simulink model "rr_arm_control"  (R2026a)
settings: Solver=VariableStepAuto  MaxStep=1E-03
InitFcn:
  | rr_arm_control_init;
values from neighbouring files (symbols this model uses):
  b1 = 0.9    [rr_arm_control_init.m]
  b2 = 0.9    [rr_arm_control_init.m]
  g = 9.81    [rr_arm_control_init.m]
  G1 = blkdiag(diag([Ixx1,Iyy1,Izz1]),m1*eye(3))    [rr_arm_control_init.m]
  G2 = blkdiag(diag([Ixx2,Iyy2,Izz2]),m2*eye(3))    [rr_arm_control_init.m]
  M1 = [ ... (first row only)    [rr_arm_control_init.m]
  M2 = [ ... (first row only)    [rr_arm_control_init.m]
  params = [Iyy1,Iyy2,m1,m2,l1,l2,b1,b2,g].'    [rr_arm_control_init.m]
  S1 = rscrew('y',[0,0,0])    [rr_arm_control_init.m]
  S2 = rscrew('y',[l1,0,0])    [rr_arm_control_init.m]
(part 1 of 2)
settings Model: Creator=marti  LastModifiedBy=marti
settings SimscapeCC: SimscapeNominalValues="[{\"value\":\"1\",\"unit\":\"A\"},{\"value\":\"1\",\"unit\":\"bar\"},{\"value\":\"1\",\"unit\":\"cm^2\"},{\"value\":\"1\",\"unit\":\"cm^3/s\"},{\"value\":\"1\",\"unit\":\"kJ/kg\"},{\"value\":\"1\",\"unit\":\"kW\"},{\"value\":\"1\",\"unit\":\"l\"},{\"value\":\"1\",\"unit\":\"N\"},{\"value\":\"1\",\"unit\":\"N*m\"},{\"value\":\"1\",\"unit\":\"V\"}]"  SimscapeLogType=none  SimscapeLogDataHistory=5000.0

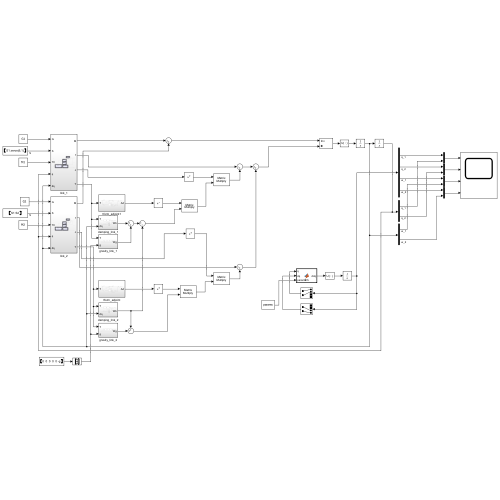
[thumbnail: Simulink's stored preview of the top-level diagram]
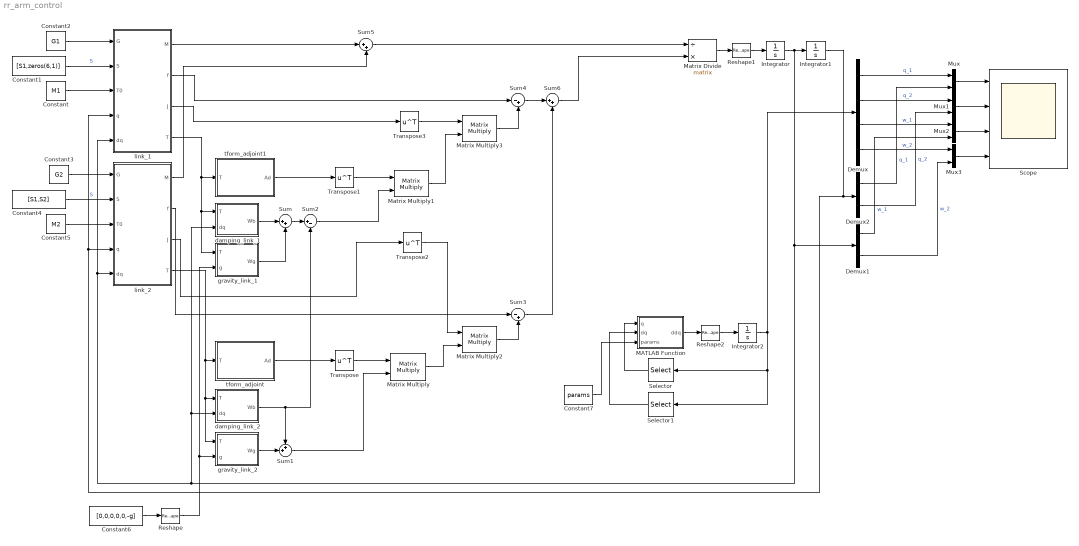
== system rr_arm_control ==
  Constant : Constant  Value=M1
  Constant1 : Constant  Value=[S1,zeros(6,1)]
  Constant2 : Constant  Value=G1
  Constant3 : Constant  Value=G2
  Constant4 : Constant  Value=[S1,S2]
  Constant5 : Constant  Value=M2
  Constant6 : Constant  Value=[0,0,0,0,0,-g]
  Constant7 : Constant  Value=params
  Demux : Demux
  Demux1 : Demux  Outputs=2
  Demux2 : Demux  Outputs=2
  Integrator : Integrator
  Integrator1 : Integrator  WrappedStateUpperValue=[pi,pi]'  WrappedStateLowerValue=-[pi,pi]'
  Integrator2 : Integrator
  MATLAB Function : MATLAB Function  TreatAsAtomicUnit=on
  Matrix Divide : Product  Inputs=/*  Multiplication=Matrix(*)
  Matrix Multiply{,1..3} (4 alike) : Product  Multiplication=Matrix(*)
  Mux{,1..3} (4 alike) : Mux  Inputs=2
  Reshape : Reshape  OutputDimensionality=Column vector (2-D)
  Reshape1 : Reshape
  Reshape2 : Reshape
  Scope : Scope  NumInputPorts=4
      settings: Title=q_1  ActiveDisplayYMinimum=-0.36221753295420889  ActiveDisplayYMaximum=3.2599577965878805  YLabel=angle (rad)
  Selector : Selector  InputPortWidth=4  IndexOptions=Index vector (dialog)  Indices=1:2  OutputSizes=1
  Selector1 : Selector  InputPortWidth=4  IndexOptions=Index vector (dialog)  Indices=3:4  OutputSizes=1
  Sum : Sum  Inputs=|++
  Sum1 : Sum  Inputs=++|
  Sum2 : Sum  Inputs=|+-
  Sum3 : Sum  Inputs=|-+
  Sum4 : Sum  Inputs=|-+
  Sum5 : Sum  Inputs=|++
  Sum6 : Sum  Inputs=|++
  Transpose{,1..3} (4 alike) : Math  Operator=transpose
  damping_link_1 : Subsystem
  damping_link_2 : Subsystem
  gravity_link_1 : Subsystem
  gravity_link_2 : Subsystem
  link_1 : Subsystem
  link_2 : Subsystem
  tform_adjoint : Subsystem
  tform_adjoint1 : Subsystem
  wires:
  Demux/1 -> Mux/1  "q_1"
  Demux2/1 -> Mux/2  "q_1"
  Demux/2 -> Mux1/1  "q_2"
  Demux2/2 -> Mux1/2  "q_2"
  Demux/3 -> Mux2/1  "w_1"
  Demux1/1 -> Mux2/2  "w_1"
  Demux/4 -> Mux3/1  "w_2"
  Demux1/2 -> Mux3/2  "w_2"
  Mux3/1 -> Scope/4
  Mux2/1 -> Scope/3
  Mux1/1 -> Scope/2
  Mux/1 -> Scope/1
  Constant2/1 -> link_1/1(G)
  Constant1/1 -> link_1/2(S)  "S"
  Constant/1 -> link_1/3(T0)
  Constant3/1 -> link_2/1(G)
  Constant4/1 -> link_2/2(S)  "S"
  Constant5/1 -> link_2/3(T0)
  Constant6/1 -> Reshape/1
  Matrix Divide/1 -> Reshape1/1
  Integrator/1 -> Integrator1/1, damping_link_2/2(dq), damping_link_1/2(dq), link_1/5(dq), link_2/5(dq), Demux1/1
  Reshape1/1 -> Integrator/1
  Integrator1/1 -> Demux2/1, link_1/4(q), link_2/4(q)
  MATLAB Function/1(ddq) -> Reshape2/1
  Reshape2/1 -> Integrator2/1
  Integrator2/1 -> Selector/1, Selector1/1, Demux/1
  Constant7/1 -> MATLAB Function/3(params)
  Selector/1 -> MATLAB Function/1(q)
  Selector1/1 -> MATLAB Function/2(dq)
  tform_adjoint/1(Ad) -> Transpose/1
  Transpose/1 -> Matrix Multiply/1
  Transpose1/1 -> Matrix Multiply1/1
  tform_adjoint1/1(Ad) -> Transpose1/1
  Transpose2/1 -> Matrix Multiply2/1
  Matrix Multiply/1 -> Matrix Multiply2/2
  Transpose3/1 -> Matrix Multiply3/1
  Matrix Multiply1/1 -> Matrix Multiply3/2
  link_1/4(T) -> gravity_link_1/1(T), damping_link_1/1(T), tform_adjoint1/1(T)
  Reshape/1 -> gravity_link_2/2(g), gravity_link_1/2(g)
  link_2/4(T) -> gravity_link_2/1(T), damping_link_2/1(T), tform_adjoint/1(T)
  damping_link_1/1(Wb) -> Sum/1
  gravity_link_1/1(Wg) -> Sum/2
  damping_link_2/1(Wb) -> Sum2/2, Sum1/1
  gravity_link_2/1(Wg) -> Sum1/2
  Sum/1 -> Sum2/1
  Sum1/1 -> Matrix Multiply/2
  link_2/3(J) -> Transpose2/1
  link_2/2(f) -> Sum3/1
  Matrix Multiply2/1 -> Sum3/2
  link_1/3(J) -> Transpose3/1
  Sum2/1 -> Matrix Multiply1/2
  Matrix Multiply3/1 -> Sum4/2
  link_1/2(f) -> Sum4/1
  link_1/1(M) -> Sum5/1
  link_2/1(M) -> Sum5/2
  Sum5/1 -> Matrix Divide/1
  Sum4/1 -> Sum6/1
  Sum3/1 -> Sum6/2
  Sum6/1 -> Matrix Divide/2

== system rr_arm_control/damping_link_1 ==
  T : Inport
  dq : Inport  Port=2
  Constant : Constant  Value=0
  Gain : Gain  Gain=-b1
  Matrix Multiply1 : Product  Multiplication=Matrix(*)
  Mux : Mux  Inputs=6
  Selector : Selector  InputPortWidth=2  IndexOptions=Index vector (dialog)  Indices=1  OutputSizes=1
  Transpose1 : Math  Operator=transpose
  tform_adjoint : Subsystem
  tform_inverse : Subsystem
  Wb : Outport
  wires:
  Matrix Multiply1/1 -> Wb/1
  tform_inverse/1(Tinv) -> tform_adjoint/1(T)
  tform_adjoint/1(Ad) -> Transpose1/1
  Transpose1/1 -> Matrix Multiply1/1
  T/1 -> tform_inverse/1(T)
  dq/1 -> Selector/1
  Selector/1 -> Gain/1
  Constant/1 -> Mux/6, Mux/5, Mux/4, Mux/3, Mux/1
  Gain/1 -> Mux/2
  Mux/1 -> Matrix Multiply1/2

== system rr_arm_control/damping_link_2 ==
  T : Inport
  dq : Inport  Port=2
  Constant : Constant  Value=0
  Gain : Gain  Gain=-b2
  Matrix Multiply1 : Product  Multiplication=Matrix(*)
  Mux : Mux  Inputs=6
  Selector : Selector  InputPortWidth=2  IndexOptions=Index vector (dialog)  Indices=2  OutputSizes=1
  Transpose1 : Math  Operator=transpose
  tform_adjoint : Subsystem
  tform_inverse : Subsystem
  Wb : Outport
  wires:
  Matrix Multiply1/1 -> Wb/1
  tform_inverse/1(Tinv) -> tform_adjoint/1(T)
  tform_adjoint/1(Ad) -> Transpose1/1
  Transpose1/1 -> Matrix Multiply1/1
  T/1 -> tform_inverse/1(T)
  dq/1 -> Selector/1
  Selector/1 -> Gain/1
  Constant/1 -> Mux/6, Mux/5, Mux/4, Mux/3, Mux/1
  Gain/1 -> Mux/2
  Mux/1 -> Matrix Multiply1/2

== system rr_arm_control/gravity_link_1 ==
  T : Inport
  g : Inport  Port=2
  Constant : Constant  Value=eye(3)
  Matrix Multiply1 : Product  Multiplication=Matrix(*)
  Selector : Selector  NumberOfDimensions=2  InputPortWidth=3  IndexOptions=Index vector (dialog),Index vector (dialog)  Indices=1:3,4  OutputSizes=1,1
  Transpose1 : Math  Operator=transpose
  tform : Subsystem
  tform_adjoint : Subsystem
  tform_inverse : Subsystem
  Wg : Outport
  wires:
  Matrix Multiply1/1 -> Wg/1
  T/1 -> Selector/1
  Selector/1 -> tform/2(p)
  Constant/1 -> tform/1(R)
  tform_inverse/1(Tinv) -> tform_adjoint/1(T)
  tform/1(T) -> tform_inverse/1(T)
  tform_adjoint/1(Ad) -> Transpose1/1
  Transpose1/1 -> Matrix Multiply1/1
  g/1 -> Matrix Multiply1/2

== system rr_arm_control/gravity_link_2 ==
  T : Inport
  g : Inport  Port=2
  Constant : Constant  Value=eye(3)
  Matrix Multiply1 : Product  Multiplication=Matrix(*)
  Selector : Selector  NumberOfDimensions=2  InputPortWidth=3  IndexOptions=Index vector (dialog),Index vector (dialog)  Indices=1:3,4  OutputSizes=1,1
  Transpose1 : Math  Operator=transpose
  tform : Subsystem
  tform_adjoint : Subsystem
  tform_inverse : Subsystem
  Wg : Outport
  wires:
  Matrix Multiply1/1 -> Wg/1
  T/1 -> Selector/1
  Selector/1 -> tform/2(p)
  Constant/1 -> tform/1(R)
  tform_inverse/1(Tinv) -> tform_adjoint/1(T)
  tform/1(T) -> tform_inverse/1(T)
  tform_adjoint/1(Ad) -> Transpose1/1
  Transpose1/1 -> Matrix Multiply1/1
  g/1 -> Matrix Multiply1/2

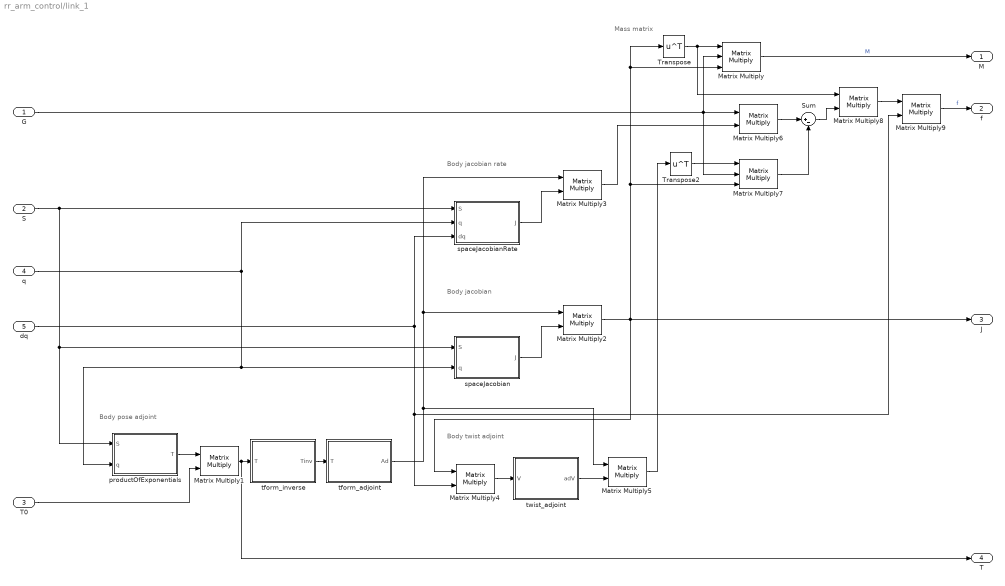
== system rr_arm_control/link_1 ==
  note: Body jacobian
  note: Body twist adjoint
  note: Mass matrix
  note: Body jacobian rate
  note: Body pose adjoint
  G : Inport
  S : Inport  Port=2
  T0 : Inport  Port=3
  q : Inport  Port=4
  dq : Inport  Port=5
  Matrix Multiply : Product  Inputs=3  Multiplication=Matrix(*)
  Matrix Multiply{1..6,8..9} (8 alike) : Product  Multiplication=Matrix(*)
  Matrix Multiply7 : Product  Inputs=3  Multiplication=Matrix(*)
  Sum : Sum  Inputs=|+-
  Transpose : Math  Operator=transpose
  Transpose2 : Math  Operator=transpose
  productOfExponentials : Subsystem  TreatAsAtomicUnit=on
  spaceJacobian : Subsystem  TreatAsAtomicUnit=on
  spaceJacobianRate : Subsystem  TreatAsAtomicUnit=on
  tform_adjoint : Subsystem
  tform_inverse : Subsystem
  twist_adjoint : Subsystem
  M : Outport
  f : Outport  Port=2
  J : Outport  Port=3
  T : Outport  Port=4
  wires:
  Matrix Multiply3/1 -> Matrix Multiply6/2
  Matrix Multiply2/1 -> Matrix Multiply7/3, Matrix Multiply/3, Transpose/1, J/1, Matrix Multiply4/1
  S/1 -> productOfExponentials/1(S), spaceJacobian/1(S), spaceJacobianRate/1(S)
  Matrix Multiply6/1 -> Sum/1
  G/1 -> Matrix Multiply6/1, Matrix Multiply7/2, Matrix Multiply/2
  twist_adjoint/1(adV) -> Matrix Multiply5/2
  Transpose/1 -> Matrix Multiply8/1, Matrix Multiply/1
  productOfExponentials/1(T) -> Matrix Multiply1/1
  spaceJacobian/1(J) -> Matrix Multiply2/2
  tform_inverse/1(Tinv) -> tform_adjoint/1(T)
  Matrix Multiply8/1 -> Matrix Multiply9/1
  tform_adjoint/1(Ad) -> Matrix Multiply3/1, Matrix Multiply2/1, Matrix Multiply5/1
  Matrix Multiply5/1 -> Transpose2/1
  q/1 -> spaceJacobian/2(q), productOfExponentials/2(q), spaceJacobianRate/2(q)
  Matrix Multiply1/1 -> T/1, tform_inverse/1(T)
  Matrix Multiply7/1 -> Sum/2
  Sum/1 -> Matrix Multiply8/2
  Matrix Multiply/1 -> M/1  "M"
  spaceJacobianRate/1(J) -> Matrix Multiply3/2
  Matrix Multiply4/1 -> twist_adjoint/1(V)
  T0/1 -> Matrix Multiply1/2
  dq/1 -> Matrix Multiply9/2, Matrix Multiply4/2, spaceJacobianRate/3(dq)
  Matrix Multiply9/1 -> f/1  "f"
  Transpose2/1 -> Matrix Multiply7/1

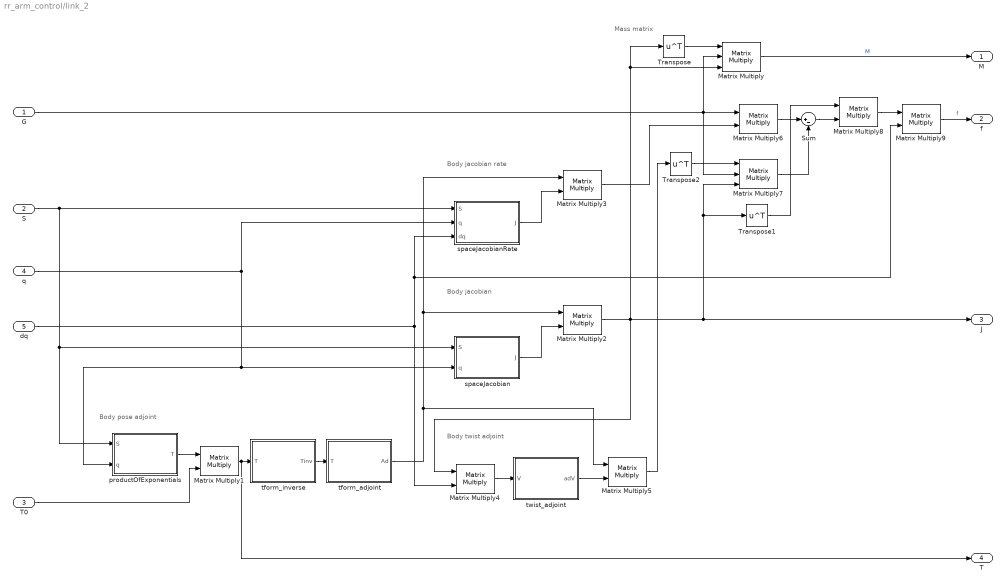
== system rr_arm_control/link_2 ==
  note: Body jacobian
  note: Body twist adjoint
  note: Mass matrix
  note: Body jacobian rate
  note: Body pose adjoint
  G : Inport
  S : Inport  Port=2
  T0 : Inport  Port=3
  q : Inport  Port=4
  dq : Inport  Port=5
  Matrix Multiply : Product  Inputs=3  Multiplication=Matrix(*)
  Matrix Multiply{1..6,8..9} (8 alike) : Product  Multiplication=Matrix(*)
  Matrix Multiply7 : Product  Inputs=3  Multiplication=Matrix(*)
  Sum : Sum  Inputs=|+-
  Transpose : Math  Operator=transpose
  Transpose1 : Math  Operator=transpose
  Transpose2 : Math  Operator=transpose
  productOfExponentials : Subsystem  TreatAsAtomicUnit=on
  spaceJacobian : Subsystem  TreatAsAtomicUnit=on
  spaceJacobianRate : Subsystem  TreatAsAtomicUnit=on
  tform_adjoint : Subsystem
  tform_inverse : Subsystem
  twist_adjoint : Subsystem
  M : Outport
  f : Outport  Port=2
  J : Outport  Port=3
  T : Outport  Port=4
  wires:
  Matrix Multiply3/1 -> Matrix Multiply6/2
  Matrix Multiply2/1 -> J/1, Transpose1/1, Matrix Multiply7/3, Matrix Multiply4/1, Matrix Multiply/3, Transpose/1
  S/1 -> productOfExponentials/1(S), spaceJacobian/1(S), spaceJacobianRate/1(S)
  Matrix Multiply6/1 -> Sum/1
  Transpose1/1 -> Matrix Multiply8/1
  G/1 -> Matrix Multiply6/1, Matrix Multiply7/2, Matrix Multiply/2
  twist_adjoint/1(adV) -> Matrix Multiply5/2
  Transpose/1 -> Matrix Multiply/1
  productOfExponentials/1(T) -> Matrix Multiply1/1
  spaceJacobian/1(J) -> Matrix Multiply2/2
  tform_inverse/1(Tinv) -> tform_adjoint/1(T)
  Matrix Multiply8/1 -> Matrix Multiply9/1
  tform_adjoint/1(Ad) -> Matrix Multiply3/1, Matrix Multiply2/1, Matrix Multiply5/1
  Matrix Multiply5/1 -> Transpose2/1
  q/1 -> spaceJacobian/2(q), productOfExponentials/2(q), spaceJacobianRate/2(q)
  Matrix Multiply1/1 -> T/1, tform_inverse/1(T)
  Matrix Multiply7/1 -> Sum/2
  Sum/1 -> Matrix Multiply8/2
  Matrix Multiply/1 -> M/1  "M"
  spaceJacobianRate/1(J) -> Matrix Multiply3/2
  Matrix Multiply4/1 -> twist_adjoint/1(V)
  T0/1 -> Matrix Multiply1/2
  dq/1 -> spaceJacobianRate/3(dq), Matrix Multiply9/2, Matrix Multiply4/2
  Matrix Multiply9/1 -> f/1  "f"
  Transpose2/1 -> Matrix Multiply7/1

== system rr_arm_control/tform_adjoint ==
  T : Inport
  Constant : Constant  Value=zeros(3)
  Matrix Concatenate : Concatenate  Mode=Multidimensional array  ConcatenateDimension=2
  Matrix Concatenate1 : Concatenate  Mode=Multidimensional array  ConcatenateDimension=2
  Matrix Concatenate2 : Concatenate  Mode=Multidimensional array
  Matrix Multiply : Product  Multiplication=Matrix(*)
  Selector : Selector  NumberOfDimensions=2  InputPortWidth=3  IndexOptions=Index vector (dialog),Index vector (dialog)  Indices=1:3,1:3  OutputSizes=1,1
  Selector1 : Selector  NumberOfDimensions=2  InputPortWidth=3  IndexOptions=Index vector (dialog),Index vector (dialog)  Indices=1:3,4  OutputSizes=1,1
  vec2skew : Subsystem
  Ad : Outport
  wires:
  Selector1/1 -> vec2skew/1(x)
  Selector/1 -> Matrix Multiply/2, Matrix Concatenate1/2, Matrix Concatenate/1
  Constant/1 -> Matrix Concatenate/2
  vec2skew/1("[x]") -> Matrix Multiply/1
  Matrix Multiply/1 -> Matrix Concatenate1/1
  Matrix Concatenate1/1 -> Matrix Concatenate2/2
  Matrix Concatenate/1 -> Matrix Concatenate2/1
  Matrix Concatenate2/1 -> Ad/1
  T/1 -> Selector1/1, Selector/1

== system rr_arm_control/tform_adjoint1 ==
  T : Inport
  Constant : Constant  Value=zeros(3)
  Matrix Concatenate : Concatenate  Mode=Multidimensional array  ConcatenateDimension=2
  Matrix Concatenate1 : Concatenate  Mode=Multidimensional array  ConcatenateDimension=2
  Matrix Concatenate2 : Concatenate  Mode=Multidimensional array
  Matrix Multiply : Product  Multiplication=Matrix(*)
  Selector : Selector  NumberOfDimensions=2  InputPortWidth=3  IndexOptions=Index vector (dialog),Index vector (dialog)  Indices=1:3,1:3  OutputSizes=1,1
  Selector1 : Selector  NumberOfDimensions=2  InputPortWidth=3  IndexOptions=Index vector (dialog),Index vector (dialog)  Indices=1:3,4  OutputSizes=1,1
  vec2skew : Subsystem
  Ad : Outport
  wires:
  Selector1/1 -> vec2skew/1(x)
  Selector/1 -> Matrix Multiply/2, Matrix Concatenate1/2, Matrix Concatenate/1
  Constant/1 -> Matrix Concatenate/2
  vec2skew/1("[x]") -> Matrix Multiply/1
  Matrix Multiply/1 -> Matrix Concatenate1/1
  Matrix Concatenate1/1 -> Matrix Concatenate2/2
  Matrix Concatenate/1 -> Matrix Concatenate2/1
  Matrix Concatenate2/1 -> Ad/1
  T/1 -> Selector1/1, Selector/1

== system rr_arm_control/damping_link_1/tform_adjoint ==
  T : Inport
  Constant : Constant  Value=zeros(3)
  Matrix Concatenate : Concatenate  Mode=Multidimensional array  ConcatenateDimension=2
  Matrix Concatenate1 : Concatenate  Mode=Multidimensional array  ConcatenateDimension=2
  Matrix Concatenate2 : Concatenate  Mode=Multidimensional array
  Matrix Multiply : Product  Multiplication=Matrix(*)
  Selector : Selector  NumberOfDimensions=2  InputPortWidth=3  IndexOptions=Index vector (dialog),Index vector (dialog)  Indices=1:3,1:3  OutputSizes=1,1
  Selector1 : Selector  NumberOfDimensions=2  InputPortWidth=3  IndexOptions=Index vector (dialog),Index vector (dialog)  Indices=1:3,4  OutputSizes=1,1
  vec2skew : Subsystem
  Ad : Outport
  wires:
  Selector1/1 -> vec2skew/1(x)
  Selector/1 -> Matrix Multiply/2, Matrix Concatenate1/2, Matrix Concatenate/1
  Constant/1 -> Matrix Concatenate/2
  vec2skew/1("[x]") -> Matrix Multiply/1
  Matrix Multiply/1 -> Matrix Concatenate1/1
  Matrix Concatenate1/1 -> Matrix Concatenate2/2
  Matrix Concatenate/1 -> Matrix Concatenate2/1
  Matrix Concatenate2/1 -> Ad/1
  T/1 -> Selector1/1, Selector/1

== system rr_arm_control/damping_link_1/tform_inverse ==
  T : Inport
  Constant : Constant  Value=[0,0,0,1]
  Gain : Gain  Gain=-1
  Matrix Concatenate : Concatenate  Mode=Multidimensional array  ConcatenateDimension=2
  Matrix Concatenate1 : Concatenate  Mode=Multidimensional array
  Matrix Multiply : Product  Multiplication=Matrix(*)
  Reshape : Reshape  OutputDimensionality=Row vector (2-D)
  Selector : Selector  NumberOfDimensions=2  InputPortWidth=3  IndexOptions=Index vector (dialog),Index vector (dialog)  Indices=1:3,1:3  OutputSizes=1,1
  Selector1 : Selector  NumberOfDimensions=2  InputPortWidth=3  IndexOptions=Index vector (dialog),Index vector (dialog)  Indices=1:3,4  OutputSizes=1,1
  Transpose : Math  Operator=transpose
  Tinv : Outport
  wires:
  T/1 -> Selector1/1, Selector/1
  Selector/1 -> Transpose/1
  Transpose/1 -> Matrix Multiply/1, Matrix Concatenate/1
  Matrix Multiply/1 -> Gain/1
  Gain/1 -> Matrix Concatenate/2
  Matrix Concatenate/1 -> Matrix Concatenate1/1
  Constant/1 -> Reshape/1
  Matrix Concatenate1/1 -> Tinv/1
  Selector1/1 -> Matrix Multiply/2
  Reshape/1 -> Matrix Concatenate1/2

== system rr_arm_control/damping_link_2/tform_adjoint ==
  T : Inport
  Constant : Constant  Value=zeros(3)
  Matrix Concatenate : Concatenate  Mode=Multidimensional array  ConcatenateDimension=2
  Matrix Concatenate1 : Concatenate  Mode=Multidimensional array  ConcatenateDimension=2
  Matrix Concatenate2 : Concatenate  Mode=Multidimensional array
  Matrix Multiply : Product  Multiplication=Matrix(*)
  Selector : Selector  NumberOfDimensions=2  InputPortWidth=3  IndexOptions=Index vector (dialog),Index vector (dialog)  Indices=1:3,1:3  OutputSizes=1,1
  Selector1 : Selector  NumberOfDimensions=2  InputPortWidth=3  IndexOptions=Index vector (dialog),Index vector (dialog)  Indices=1:3,4  OutputSizes=1,1
  vec2skew : Subsystem
  Ad : Outport
  wires:
  Selector1/1 -> vec2skew/1(x)
  Selector/1 -> Matrix Multiply/2, Matrix Concatenate1/2, Matrix Concatenate/1
  Constant/1 -> Matrix Concatenate/2
  vec2skew/1("[x]") -> Matrix Multiply/1
  Matrix Multiply/1 -> Matrix Concatenate1/1
  Matrix Concatenate1/1 -> Matrix Concatenate2/2
  Matrix Concatenate/1 -> Matrix Concatenate2/1
  Matrix Concatenate2/1 -> Ad/1
  T/1 -> Selector1/1, Selector/1

== system rr_arm_control/damping_link_2/tform_inverse ==
  T : Inport
  Constant : Constant  Value=[0,0,0,1]
  Gain : Gain  Gain=-1
  Matrix Concatenate : Concatenate  Mode=Multidimensional array  ConcatenateDimension=2
  Matrix Concatenate1 : Concatenate  Mode=Multidimensional array
  Matrix Multiply : Product  Multiplication=Matrix(*)
  Reshape : Reshape  OutputDimensionality=Row vector (2-D)
  Selector : Selector  NumberOfDimensions=2  InputPortWidth=3  IndexOptions=Index vector (dialog),Index vector (dialog)  Indices=1:3,1:3  OutputSizes=1,1
  Selector1 : Selector  NumberOfDimensions=2  InputPortWidth=3  IndexOptions=Index vector (dialog),Index vector (dialog)  Indices=1:3,4  OutputSizes=1,1
  Transpose : Math  Operator=transpose
  Tinv : Outport
  wires:
  T/1 -> Selector1/1, Selector/1
  Selector/1 -> Transpose/1
  Transpose/1 -> Matrix Multiply/1, Matrix Concatenate/1
  Matrix Multiply/1 -> Gain/1
  Gain/1 -> Matrix Concatenate/2
  Matrix Concatenate/1 -> Matrix Concatenate1/1
  Constant/1 -> Reshape/1
  Matrix Concatenate1/1 -> Tinv/1
  Selector1/1 -> Matrix Multiply/2
  Reshape/1 -> Matrix Concatenate1/2

== system rr_arm_control/gravity_link_1/tform ==
  R : Inport
  p : Inport  Port=2
  Constant : Constant  Value=[0,0,0,1]
  Matrix Concatenate : Concatenate  Mode=Multidimensional array  ConcatenateDimension=2
  Matrix Concatenate2 : Concatenate  Mode=Multidimensional array
  Reshape : Reshape  OutputDimensionality=Row vector (2-D)
  T : Outport
  wires:
  p/1 -> Matrix Concatenate/2
  Constant/1 -> Reshape/1
  Matrix Concatenate/1 -> Matrix Concatenate2/1
  Matrix Concatenate2/1 -> T/1
  R/1 -> Matrix Concatenate/1
  Reshape/1 -> Matrix Concatenate2/2

== system rr_arm_control/gravity_link_1/tform_adjoint ==
  T : Inport
  Constant : Constant  Value=zeros(3)
  Matrix Concatenate : Concatenate  Mode=Multidimensional array  ConcatenateDimension=2
  Matrix Concatenate1 : Concatenate  Mode=Multidimensional array  ConcatenateDimension=2
  Matrix Concatenate2 : Concatenate  Mode=Multidimensional array
  Matrix Multiply : Product  Multiplication=Matrix(*)
  Selector : Selector  NumberOfDimensions=2  InputPortWidth=3  IndexOptions=Index vector (dialog),Index vector (dialog)  Indices=1:3,1:3  OutputSizes=1,1
  Selector1 : Selector  NumberOfDimensions=2  InputPortWidth=3  IndexOptions=Index vector (dialog),Index vector (dialog)  Indices=1:3,4  OutputSizes=1,1
  vec2skew : Subsystem
  Ad : Outport
  wires:
  Selector1/1 -> vec2skew/1(x)
  Selector/1 -> Matrix Multiply/2, Matrix Concatenate1/2, Matrix Concatenate/1
  Constant/1 -> Matrix Concatenate/2
  vec2skew/1("[x]") -> Matrix Multiply/1
  Matrix Multiply/1 -> Matrix Concatenate1/1
  Matrix Concatenate1/1 -> Matrix Concatenate2/2
  Matrix Concatenate/1 -> Matrix Concatenate2/1
  Matrix Concatenate2/1 -> Ad/1
  T/1 -> Selector1/1, Selector/1

== system rr_arm_control/gravity_link_1/tform_inverse ==
  T : Inport
  Constant : Constant  Value=[0,0,0,1]
  Gain : Gain  Gain=-1
  Matrix Concatenate : Concatenate  Mode=Multidimensional array  ConcatenateDimension=2
  Matrix Concatenate1 : Concatenate  Mode=Multidimensional array
  Matrix Multiply : Product  Multiplication=Matrix(*)
  Reshape : Reshape  OutputDimensionality=Row vector (2-D)
  Selector : Selector  NumberOfDimensions=2  InputPortWidth=3  IndexOptions=Index vector (dialog),Index vector (dialog)  Indices=1:3,1:3  OutputSizes=1,1
  Selector1 : Selector  NumberOfDimensions=2  InputPortWidth=3  IndexOptions=Index vector (dialog),Index vector (dialog)  Indices=1:3,4  OutputSizes=1,1
  Transpose : Math  Operator=transpose
  Tinv : Outport
  wires:
  T/1 -> Selector1/1, Selector/1
  Selector/1 -> Transpose/1
  Transpose/1 -> Matrix Multiply/1, Matrix Concatenate/1
  Matrix Multiply/1 -> Gain/1
  Gain/1 -> Matrix Concatenate/2
  Matrix Concatenate/1 -> Matrix Concatenate1/1
  Constant/1 -> Reshape/1
  Matrix Concatenate1/1 -> Tinv/1
  Selector1/1 -> Matrix Multiply/2
  Reshape/1 -> Matrix Concatenate1/2

== system rr_arm_control/gravity_link_2/tform ==
  R : Inport
  p : Inport  Port=2
  Constant : Constant  Value=[0,0,0,1]
  Matrix Concatenate : Concatenate  Mode=Multidimensional array  ConcatenateDimension=2
  Matrix Concatenate2 : Concatenate  Mode=Multidimensional array
  Reshape : Reshape  OutputDimensionality=Row vector (2-D)
  T : Outport
  wires:
  p/1 -> Matrix Concatenate/2
  Constant/1 -> Reshape/1
  Matrix Concatenate/1 -> Matrix Concatenate2/1
  Matrix Concatenate2/1 -> T/1
  R/1 -> Matrix Concatenate/1
  Reshape/1 -> Matrix Concatenate2/2

== system rr_arm_control/gravity_link_2/tform_adjoint ==
  T : Inport
  Constant : Constant  Value=zeros(3)
  Matrix Concatenate : Concatenate  Mode=Multidimensional array  ConcatenateDimension=2
  Matrix Concatenate1 : Concatenate  Mode=Multidimensional array  ConcatenateDimension=2
  Matrix Concatenate2 : Concatenate  Mode=Multidimensional array
  Matrix Multiply : Product  Multiplication=Matrix(*)
  Selector : Selector  NumberOfDimensions=2  InputPortWidth=3  IndexOptions=Index vector (dialog),Index vector (dialog)  Indices=1:3,1:3  OutputSizes=1,1
  Selector1 : Selector  NumberOfDimensions=2  InputPortWidth=3  IndexOptions=Index vector (dialog),Index vector (dialog)  Indices=1:3,4  OutputSizes=1,1
  vec2skew : Subsystem
  Ad : Outport
  wires:
  Selector1/1 -> vec2skew/1(x)
  Selector/1 -> Matrix Multiply/2, Matrix Concatenate1/2, Matrix Concatenate/1
  Constant/1 -> Matrix Concatenate/2
  vec2skew/1("[x]") -> Matrix Multiply/1
  Matrix Multiply/1 -> Matrix Concatenate1/1
  Matrix Concatenate1/1 -> Matrix Concatenate2/2
  Matrix Concatenate/1 -> Matrix Concatenate2/1
  Matrix Concatenate2/1 -> Ad/1
  T/1 -> Selector1/1, Selector/1

== system rr_arm_control/gravity_link_2/tform_inverse ==
  T : Inport
  Constant : Constant  Value=[0,0,0,1]
  Gain : Gain  Gain=-1
  Matrix Concatenate : Concatenate  Mode=Multidimensional array  ConcatenateDimension=2
  Matrix Concatenate1 : Concatenate  Mode=Multidimensional array
  Matrix Multiply : Product  Multiplication=Matrix(*)
  Reshape : Reshape  OutputDimensionality=Row vector (2-D)
  Selector : Selector  NumberOfDimensions=2  InputPortWidth=3  IndexOptions=Index vector (dialog),Index vector (dialog)  Indices=1:3,1:3  OutputSizes=1,1
  Selector1 : Selector  NumberOfDimensions=2  InputPortWidth=3  IndexOptions=Index vector (dialog),Index vector (dialog)  Indices=1:3,4  OutputSizes=1,1
  Transpose : Math  Operator=transpose
  Tinv : Outport
  wires:
  T/1 -> Selector1/1, Selector/1
  Selector/1 -> Transpose/1
  Transpose/1 -> Matrix Multiply/1, Matrix Concatenate/1
  Matrix Multiply/1 -> Gain/1
  Gain/1 -> Matrix Concatenate/2
  Matrix Concatenate/1 -> Matrix Concatenate1/1
  Constant/1 -> Reshape/1
  Matrix Concatenate1/1 -> Tinv/1
  Selector1/1 -> Matrix Multiply/2
  Reshape/1 -> Matrix Concatenate1/2

== system rr_arm_control/link_1/productOfExponentials ==
  S : Inport
  q : Inport  Port=2
  For Iterator : ForIterator  ResetStates=reset  IterationSource=external
  Matrix Multiply : Product  Multiplication=Matrix(*)
  Memory : Memory  InitialCondition=eye(4)  InheritSampleTime=on
  Probe Dimension : Probe  ProbeWidth=off  ProbeSampleTime=off  ProbeComplexSignal=off  ProbeSignalDimensions=on
  Reshape : Reshape  OutputDimensionality=Column vector (2-D)
  Selector : Selector  NumberOfDimensions=2  InputPortWidth=3  IndexOptions=Select all,Index vector (port)  Indices=[1 3],1  OutputSizes=1,1
  Selector1 : Selector  NumberOfDimensions=2  InputPortWidth=3  IndexOptions=Index vector (port),Select all  Indices=[1 3],1  OutputSizes=1,1
  Subsystem1 : Subsystem
  T : Outport
  wires:
  For Iterator/1 -> Selector1/2, Selector/2
  q/1 -> Reshape/1, Probe Dimension/1
  Probe Dimension/1 -> For Iterator/1
  S/1 -> Selector/1
  Selector/1 -> Subsystem1/1(S)
  Reshape/1 -> Selector1/1
  Selector1/1 -> Subsystem1/2(q)
  Subsystem1/1(T) -> Matrix Multiply/2
  Matrix Multiply/1 -> Memory/1, T/1
  Memory/1 -> Matrix Multiply/1

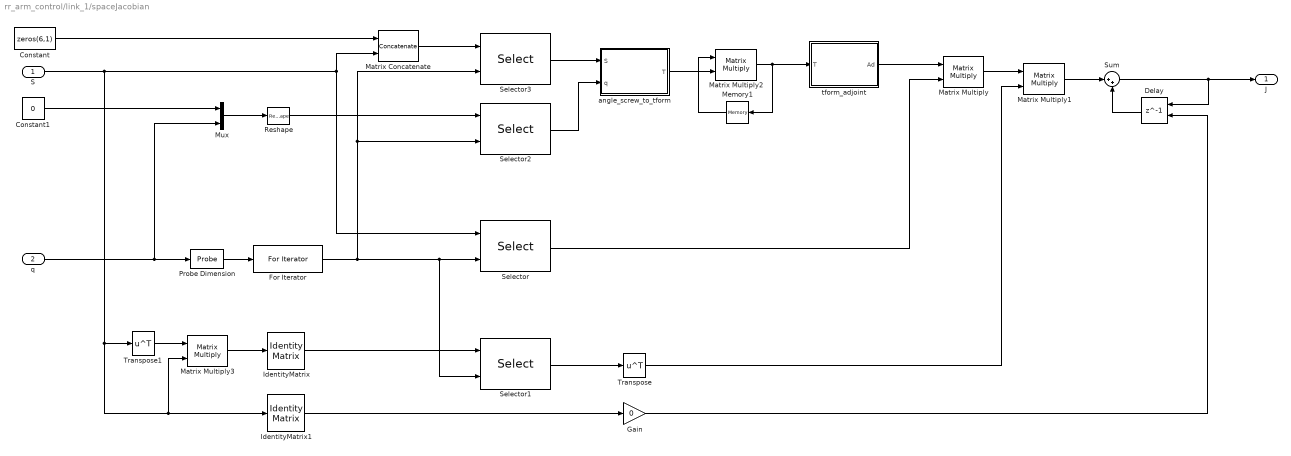
== system rr_arm_control/link_1/spaceJacobian ==
  S : Inport
  q : Inport  Port=2
  Constant : Constant  Value=zeros(6,1)
  Constant1 : Constant  Value=0
  Delay : Delay  DelayLength=1  InitialConditionSource=Input port
      settings: InputPortMap=u0,p4
  For Iterator : ForIterator  ResetStates=reset  IterationSource=external  IterationLimit=4
  Gain : Gain  Gain=0
  IdentityMatrix : IdentityMatrix  InheritOutputPortAttributes=on
  IdentityMatrix1 : IdentityMatrix  InheritOutputPortAttributes=on
  Matrix Concatenate : Concatenate  Mode=Multidimensional array  ConcatenateDimension=2
  Matrix Multiply{,1..3} (4 alike) : Product  Multiplication=Matrix(*)
  Memory1 : Memory  InitialCondition=eye(4)  InheritSampleTime=on
  Mux : Mux  Inputs=2
  Probe Dimension : Probe  ProbeWidth=off  ProbeSampleTime=off  ProbeComplexSignal=off  ProbeSignalDimensions=on
  Reshape : Reshape  OutputDimensionality=Column vector (2-D)
  Selector : Selector  NumberOfDimensions=2  InputPortWidth=3  IndexOptions=Select all,Index vector (port)  Indices=[1 3],1  OutputSizes=1,1
  Selector1 : Selector  NumberOfDimensions=2  InputPortWidth=3  IndexOptions=Select all,Index vector (port)  Indices=[1 3],1  OutputSizes=1,1
  Selector2 : Selector  NumberOfDimensions=2  InputPortWidth=3  IndexOptions=Index vector (port),Select all  Indices=[1 3],1  OutputSizes=1,1
  Selector3 : Selector  NumberOfDimensions=2  InputPortWidth=3  IndexOptions=Select all,Index vector (port)  Indices=[1 3],1  OutputSizes=1,1
  Sum : Sum  Inputs=|++
  Transpose : Math  Operator=transpose
  Transpose1 : Math  Operator=transpose
  angle_screw_to_tform : Subsystem
  tform_adjoint : Subsystem
  J : Outport
  wires:
  S/1 -> Matrix Concatenate/2, Selector/1, IdentityMatrix1/1, Matrix Multiply3/2, Transpose1/1
  Matrix Multiply1/1 -> Sum/1
  Sum/1 -> Delay/1, J/1
  tform_adjoint/1(Ad) -> Matrix Multiply/1
  Selector/1 -> Matrix Multiply/2
  For Iterator/1 -> Selector1/2, Selector/2, Selector3/2, Selector2/2
  Matrix Multiply/1 -> Matrix Multiply1/1
  Transpose/1 -> Matrix Multiply1/2
  angle_screw_to_tform/1(T) -> Matrix Multiply2/2
  Matrix Multiply2/1 -> tform_adjoint/1(T), Memory1/1
  Memory1/1 -> Matrix Multiply2/1
  Selector2/1 -> angle_screw_to_tform/2(q)
  Selector3/1 -> angle_screw_to_tform/1(S)
  IdentityMatrix/1 -> Selector1/1
  Selector1/1 -> Transpose/1
  q/1 -> Mux/2, Probe Dimension/1
  Matrix Multiply3/1 -> IdentityMatrix/1
  Transpose1/1 -> Matrix Multiply3/1
  IdentityMatrix1/1 -> Gain/1
  Gain/1 -> Delay/2
  Delay/1 -> Sum/2
  Probe Dimension/1 -> For Iterator/1
  Mux/1 -> Reshape/1
  Constant1/1 -> Mux/1
  Reshape/1 -> Selector2/1
  Matrix Concatenate/1 -> Selector3/1
  Constant/1 -> Matrix Concatenate/1

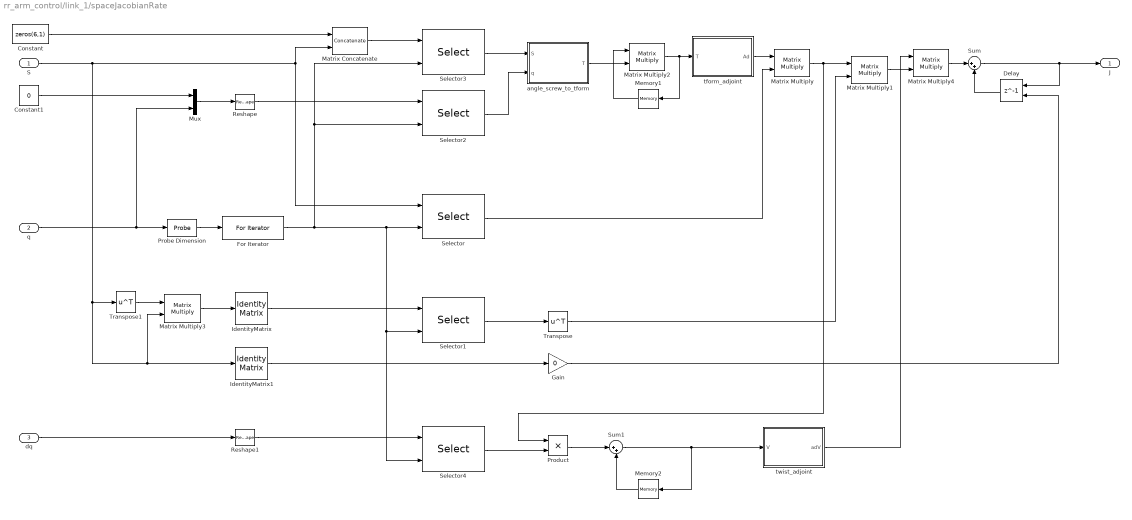
== system rr_arm_control/link_1/spaceJacobianRate ==
  S : Inport
  q : Inport  Port=2
  dq : Inport  Port=3
  Constant : Constant  Value=zeros(6,1)
  Constant1 : Constant  Value=0
  Delay : Delay  DelayLength=1  InitialConditionSource=Input port
      settings: InputPortMap=u0,p4
  For Iterator : ForIterator  ResetStates=reset  IterationSource=external  IterationLimit=4
  Gain : Gain  Gain=0
  IdentityMatrix : IdentityMatrix  InheritOutputPortAttributes=on
  IdentityMatrix1 : IdentityMatrix  InheritOutputPortAttributes=on
  Matrix Concatenate : Concatenate  Mode=Multidimensional array  ConcatenateDimension=2
  Matrix Multiply{,1..4} (5 alike) : Product  Multiplication=Matrix(*)
  Memory1 : Memory  InitialCondition=eye(4)  InheritSampleTime=on
  Memory2 : Memory  InitialCondition=zeros(6,1)  InheritSampleTime=on
  Mux : Mux  Inputs=2
  Probe Dimension : Probe  ProbeWidth=off  ProbeSampleTime=off  ProbeComplexSignal=off  ProbeSignalDimensions=on
  Product : Product
  Reshape : Reshape  OutputDimensionality=Column vector (2-D)
  Reshape1 : Reshape  OutputDimensionality=Column vector (2-D)
  Selector : Selector  NumberOfDimensions=2  InputPortWidth=3  IndexOptions=Select all,Index vector (port)  Indices=[1 3],1  OutputSizes=1,1
  Selector1 : Selector  NumberOfDimensions=2  InputPortWidth=3  IndexOptions=Select all,Index vector (port)  Indices=[1 3],1  OutputSizes=1,1
  Selector2 : Selector  NumberOfDimensions=2  InputPortWidth=3  IndexOptions=Index vector (port),Select all  Indices=[1 3],1  OutputSizes=1,1
  Selector3 : Selector  NumberOfDimensions=2  InputPortWidth=3  IndexOptions=Select all,Index vector (port)  Indices=[1 3],1  OutputSizes=1,1
  Selector4 : Selector  NumberOfDimensions=2  InputPortWidth=3  IndexOptions=Index vector (port),Select all  Indices=[1 3],1  OutputSizes=1,1
  Sum : Sum  Inputs=|++
  Sum1 : Sum  Inputs=|++
  Transpose : Math  Operator=transpose
  Transpose1 : Math  Operator=transpose
  angle_screw_to_tform : Subsystem
  tform_adjoint : Subsystem
  twist_adjoint : Subsystem
  J : Outport
  wires:
  S/1 -> Matrix Concatenate/2, Selector/1, IdentityMatrix1/1, Matrix Multiply3/2, Transpose1/1
  Sum/1 -> Delay/1, J/1
  tform_adjoint/1(Ad) -> Matrix Multiply/1
  Selector/1 -> Matrix Multiply/2
  For Iterator/1 -> Selector4/2, Selector1/2, Selector/2, Selector3/2, Selector2/2
  Matrix Multiply/1 -> Product/1, Matrix Multiply1/1
  Transpose/1 -> Matrix Multiply1/2
  angle_screw_to_tform/1(T) -> Matrix Multiply2/2
  Matrix Multiply2/1 -> tform_adjoint/1(T), Memory1/1
  Memory1/1 -> Matrix Multiply2/1
  Selector2/1 -> angle_screw_to_tform/2(q)
  Selector3/1 -> angle_screw_to_tform/1(S)
  IdentityMatrix/1 -> Selector1/1
  Selector1/1 -> Transpose/1
  q/1 -> Mux/2, Probe Dimension/1
  Matrix Multiply3/1 -> IdentityMatrix/1
  Transpose1/1 -> Matrix Multiply3/1
  IdentityMatrix1/1 -> Gain/1
  Gain/1 -> Delay/2
  Delay/1 -> Sum/2
  Probe Dimension/1 -> For Iterator/1
  Mux/1 -> Reshape/1
  Constant1/1 -> Mux/1
  Reshape/1 -> Selector2/1
  Matrix Concatenate/1 -> Selector3/1
  Constant/1 -> Matrix Concatenate/1
  Matrix Multiply1/1 -> Matrix Multiply4/2
  Matrix Multiply4/1 -> Sum/1
  dq/1 -> Reshape1/1
  Reshape1/1 -> Selector4/1
  Selector4/1 -> Product/2
  Product/1 -> Sum1/1
  Memory2/1 -> Sum1/2
  Sum1/1 -> Memory2/1, twist_adjoint/1(V)
  twist_adjoint/1(adV) -> Matrix Multiply4/1

== system rr_arm_control/link_1/tform_adjoint ==
  T : Inport
  Constant : Constant  Value=zeros(3)
  Matrix Concatenate : Concatenate  Mode=Multidimensional array  ConcatenateDimension=2
  Matrix Concatenate1 : Concatenate  Mode=Multidimensional array  ConcatenateDimension=2
  Matrix Concatenate2 : Concatenate  Mode=Multidimensional array
  Matrix Multiply : Product  Multiplication=Matrix(*)
  Selector : Selector  NumberOfDimensions=2  InputPortWidth=3  IndexOptions=Index vector (dialog),Index vector (dialog)  Indices=1:3,1:3  OutputSizes=1,1
  Selector1 : Selector  NumberOfDimensions=2  InputPortWidth=3  IndexOptions=Index vector (dialog),Index vector (dialog)  Indices=1:3,4  OutputSizes=1,1
  vec2skew : Subsystem
  Ad : Outport
  wires:
  Selector1/1 -> vec2skew/1(x)
  Selector/1 -> Matrix Multiply/2, Matrix Concatenate1/2, Matrix Concatenate/1
  Constant/1 -> Matrix Concatenate/2
  vec2skew/1("[x]") -> Matrix Multiply/1
  Matrix Multiply/1 -> Matrix Concatenate1/1
  Matrix Concatenate1/1 -> Matrix Concatenate2/2
  Matrix Concatenate/1 -> Matrix Concatenate2/1
  Matrix Concatenate2/1 -> Ad/1
  T/1 -> Selector1/1, Selector/1

== system rr_arm_control/link_1/tform_inverse ==
  T : Inport
  Constant : Constant  Value=[0,0,0,1]
  Gain : Gain  Gain=-1
  Matrix Concatenate : Concatenate  Mode=Multidimensional array  ConcatenateDimension=2
  Matrix Concatenate1 : Concatenate  Mode=Multidimensional array
  Matrix Multiply : Product  Multiplication=Matrix(*)
  Reshape : Reshape  OutputDimensionality=Row vector (2-D)
  Selector : Selector  NumberOfDimensions=2  InputPortWidth=3  IndexOptions=Index vector (dialog),Index vector (dialog)  Indices=1:3,1:3  OutputSizes=1,1
  Selector1 : Selector  NumberOfDimensions=2  InputPortWidth=3  IndexOptions=Index vector (dialog),Index vector (dialog)  Indices=1:3,4  OutputSizes=1,1
  Transpose : Math  Operator=transpose
  Tinv : Outport
  wires:
  T/1 -> Selector1/1, Selector/1
  Selector/1 -> Transpose/1
  Transpose/1 -> Matrix Multiply/1, Matrix Concatenate/1
  Matrix Multiply/1 -> Gain/1
  Gain/1 -> Matrix Concatenate/2
  Matrix Concatenate/1 -> Matrix Concatenate1/1
  Constant/1 -> Reshape/1
  Matrix Concatenate1/1 -> Tinv/1
  Selector1/1 -> Matrix Multiply/2
  Reshape/1 -> Matrix Concatenate1/2

== system rr_arm_control/link_1/twist_adjoint ==
  V : Inport
  Constant : Constant  Value=zeros(3)
  Matrix Concatenate : Concatenate  Mode=Multidimensional array  ConcatenateDimension=2
  Matrix Concatenate1 : Concatenate  Mode=Multidimensional array  ConcatenateDimension=2
  Matrix Concatenate2 : Concatenate  Mode=Multidimensional array
  Selector : Selector  InputPortWidth=6  IndexOptions=Index vector (dialog)  Indices=1:3  OutputSizes=1
  Selector1 : Selector  InputPortWidth=6  IndexOptions=Index vector (dialog)  Indices=4:6  OutputSizes=1
  "[v]" : Subsystem
  "[w]" : Subsystem
  adV : Outport
  wires:
  Selector/1 -> "[w]"/1(x)
  Constant/1 -> Matrix Concatenate/2
  Matrix Concatenate1/1 -> Matrix Concatenate2/2
  Matrix Concatenate/1 -> Matrix Concatenate2/1
  Matrix Concatenate2/1 -> adV/1
  V/1 -> Selector1/1, Selector/1
  "[w]"/1("[x]") -> Matrix Concatenate1/2, Matrix Concatenate/1
  Selector1/1 -> "[v]"/1(x)
  "[v]"/1("[x]") -> Matrix Concatenate1/1

== system rr_arm_control/link_2/productOfExponentials ==
  S : Inport
  q : Inport  Port=2
  For Iterator : ForIterator  ResetStates=reset  IterationSource=external
  Matrix Multiply : Product  Multiplication=Matrix(*)
  Memory : Memory  InitialCondition=eye(4)  InheritSampleTime=on
  Probe Dimension : Probe  ProbeWidth=off  ProbeSampleTime=off  ProbeComplexSignal=off  ProbeSignalDimensions=on
  Reshape : Reshape  OutputDimensionality=Column vector (2-D)
  Selector : Selector  NumberOfDimensions=2  InputPortWidth=3  IndexOptions=Select all,Index vector (port)  Indices=[1 3],1  OutputSizes=1,1
  Selector1 : Selector  NumberOfDimensions=2  InputPortWidth=3  IndexOptions=Index vector (port),Select all  Indices=[1 3],1  OutputSizes=1,1
  Subsystem1 : Subsystem
  T : Outport
  wires:
  For Iterator/1 -> Selector1/2, Selector/2
  q/1 -> Reshape/1, Probe Dimension/1
  Probe Dimension/1 -> For Iterator/1
  S/1 -> Selector/1
  Selector/1 -> Subsystem1/1(S)
  Reshape/1 -> Selector1/1
  Selector1/1 -> Subsystem1/2(q)
  Subsystem1/1(T) -> Matrix Multiply/2
  Matrix Multiply/1 -> Memory/1, T/1
  Memory/1 -> Matrix Multiply/1

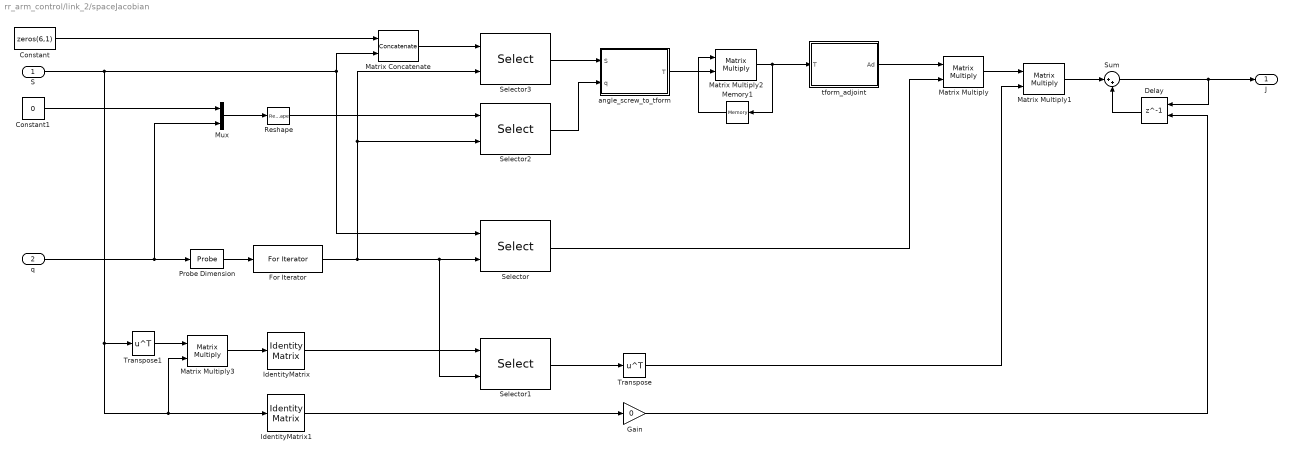
== system rr_arm_control/link_2/spaceJacobian ==
  S : Inport
  q : Inport  Port=2
  Constant : Constant  Value=zeros(6,1)
  Constant1 : Constant  Value=0
  Delay : Delay  DelayLength=1  InitialConditionSource=Input port
      settings: InputPortMap=u0,p4
  For Iterator : ForIterator  ResetStates=reset  IterationSource=external  IterationLimit=4
  Gain : Gain  Gain=0
  IdentityMatrix : IdentityMatrix  InheritOutputPortAttributes=on
  IdentityMatrix1 : IdentityMatrix  InheritOutputPortAttributes=on
  Matrix Concatenate : Concatenate  Mode=Multidimensional array  ConcatenateDimension=2
  Matrix Multiply{,1..3} (4 alike) : Product  Multiplication=Matrix(*)
  Memory1 : Memory  InitialCondition=eye(4)  InheritSampleTime=on
  Mux : Mux  Inputs=2
  Probe Dimension : Probe  ProbeWidth=off  ProbeSampleTime=off  ProbeComplexSignal=off  ProbeSignalDimensions=on
  Reshape : Reshape  OutputDimensionality=Column vector (2-D)
  Selector : Selector  NumberOfDimensions=2  InputPortWidth=3  IndexOptions=Select all,Index vector (port)  Indices=[1 3],1  OutputSizes=1,1
  Selector1 : Selector  NumberOfDimensions=2  InputPortWidth=3  IndexOptions=Select all,Index vector (port)  Indices=[1 3],1  OutputSizes=1,1
  Selector2 : Selector  NumberOfDimensions=2  InputPortWidth=3  IndexOptions=Index vector (port),Select all  Indices=[1 3],1  OutputSizes=1,1
  Selector3 : Selector  NumberOfDimensions=2  InputPortWidth=3  IndexOptions=Select all,Index vector (port)  Indices=[1 3],1  OutputSizes=1,1
  Sum : Sum  Inputs=|++
  Transpose : Math  Operator=transpose
  Transpose1 : Math  Operator=transpose
  angle_screw_to_tform : Subsystem
  tform_adjoint : Subsystem
  J : Outport
  wires:
  S/1 -> Matrix Concatenate/2, Selector/1, IdentityMatrix1/1, Matrix Multiply3/2, Transpose1/1
  Matrix Multiply1/1 -> Sum/1
  Sum/1 -> Delay/1, J/1
  tform_adjoint/1(Ad) -> Matrix Multiply/1
  Selector/1 -> Matrix Multiply/2
  For Iterator/1 -> Selector1/2, Selector/2, Selector3/2, Selector2/2
  Matrix Multiply/1 -> Matrix Multiply1/1
  Transpose/1 -> Matrix Multiply1/2
  angle_screw_to_tform/1(T) -> Matrix Multiply2/2
  Matrix Multiply2/1 -> tform_adjoint/1(T), Memory1/1
  Memory1/1 -> Matrix Multiply2/1
  Selector2/1 -> angle_screw_to_tform/2(q)
  Selector3/1 -> angle_screw_to_tform/1(S)
  IdentityMatrix/1 -> Selector1/1
  Selector1/1 -> Transpose/1
  q/1 -> Mux/2, Probe Dimension/1
  Matrix Multiply3/1 -> IdentityMatrix/1
  Transpose1/1 -> Matrix Multiply3/1
  IdentityMatrix1/1 -> Gain/1
  Gain/1 -> Delay/2
  Delay/1 -> Sum/2
  Probe Dimension/1 -> For Iterator/1
  Mux/1 -> Reshape/1
  Constant1/1 -> Mux/1
  Reshape/1 -> Selector2/1
  Matrix Concatenate/1 -> Selector3/1
  Constant/1 -> Matrix Concatenate/1

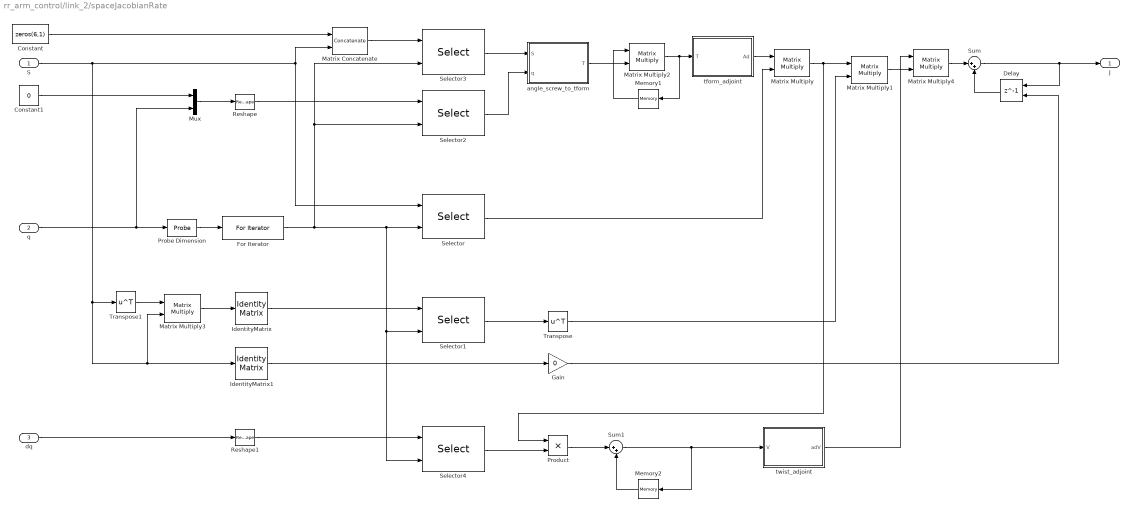
== system rr_arm_control/link_2/spaceJacobianRate ==
  S : Inport
  q : Inport  Port=2
  dq : Inport  Port=3
  Constant : Constant  Value=zeros(6,1)
  Constant1 : Constant  Value=0
  Delay : Delay  DelayLength=1  InitialConditionSource=Input port
      settings: InputPortMap=u0,p4
  For Iterator : ForIterator  ResetStates=reset  IterationSource=external  IterationLimit=4
  Gain : Gain  Gain=0
  IdentityMatrix : IdentityMatrix  InheritOutputPortAttributes=on
  IdentityMatrix1 : IdentityMatrix  InheritOutputPortAttributes=on
  Matrix Concatenate : Concatenate  Mode=Multidimensional array  ConcatenateDimension=2
  Matrix Multiply{,1..4} (5 alike) : Product  Multiplication=Matrix(*)
  Memory1 : Memory  InitialCondition=eye(4)  InheritSampleTime=on
  Memory2 : Memory  InitialCondition=zeros(6,1)  InheritSampleTime=on
  Mux : Mux  Inputs=2
  Probe Dimension : Probe  ProbeWidth=off  ProbeSampleTime=off  ProbeComplexSignal=off  ProbeSignalDimensions=on
  Product : Product
  Reshape : Reshape  OutputDimensionality=Column vector (2-D)
  Reshape1 : Reshape  OutputDimensionality=Column vector (2-D)
  Selector : Selector  NumberOfDimensions=2  InputPortWidth=3  IndexOptions=Select all,Index vector (port)  Indices=[1 3],1  OutputSizes=1,1
  Selector1 : Selector  NumberOfDimensions=2  InputPortWidth=3  IndexOptions=Select all,Index vector (port)  Indices=[1 3],1  OutputSizes=1,1
  Selector2 : Selector  NumberOfDimensions=2  InputPortWidth=3  IndexOptions=Index vector (port),Select all  Indices=[1 3],1  OutputSizes=1,1
  Selector3 : Selector  NumberOfDimensions=2  InputPortWidth=3  IndexOptions=Select all,Index vector (port)  Indices=[1 3],1  OutputSizes=1,1
  Selector4 : Selector  NumberOfDimensions=2  InputPortWidth=3  IndexOptions=Index vector (port),Select all  Indices=[1 3],1  OutputSizes=1,1
  Sum : Sum  Inputs=|++
  Sum1 : Sum  Inputs=|++
  Transpose : Math  Operator=transpose
  Transpose1 : Math  Operator=transpose
  angle_screw_to_tform : Subsystem
  tform_adjoint : Subsystem
  twist_adjoint : Subsystem
  J : Outport
  wires:
  S/1 -> Matrix Concatenate/2, Selector/1, IdentityMatrix1/1, Matrix Multiply3/2, Transpose1/1
  Sum/1 -> Delay/1, J/1
  tform_adjoint/1(Ad) -> Matrix Multiply/1
  Selector/1 -> Matrix Multiply/2
  For Iterator/1 -> Selector4/2, Selector1/2, Selector/2, Selector3/2, Selector2/2
  Matrix Multiply/1 -> Product/1, Matrix Multiply1/1
  Transpose/1 -> Matrix Multiply1/2
  angle_screw_to_tform/1(T) -> Matrix Multiply2/2
  Matrix Multiply2/1 -> tform_adjoint/1(T), Memory1/1
  Memory1/1 -> Matrix Multiply2/1
  Selector2/1 -> angle_screw_to_tform/2(q)
  Selector3/1 -> angle_screw_to_tform/1(S)
  IdentityMatrix/1 -> Selector1/1
  Selector1/1 -> Transpose/1
  q/1 -> Mux/2, Probe Dimension/1
  Matrix Multiply3/1 -> IdentityMatrix/1
  Transpose1/1 -> Matrix Multiply3/1
  IdentityMatrix1/1 -> Gain/1
  Gain/1 -> Delay/2
  Delay/1 -> Sum/2
  Probe Dimension/1 -> For Iterator/1
  Mux/1 -> Reshape/1
  Constant1/1 -> Mux/1
  Reshape/1 -> Selector2/1
  Matrix Concatenate/1 -> Selector3/1
  Constant/1 -> Matrix Concatenate/1
  Matrix Multiply1/1 -> Matrix Multiply4/2
  Matrix Multiply4/1 -> Sum/1
  dq/1 -> Reshape1/1
  Reshape1/1 -> Selector4/1
  Selector4/1 -> Product/2
  Product/1 -> Sum1/1
  Memory2/1 -> Sum1/2
  Sum1/1 -> Memory2/1, twist_adjoint/1(V)
  twist_adjoint/1(adV) -> Matrix Multiply4/1

== system rr_arm_control/link_2/tform_adjoint ==
  T : Inport
  Constant : Constant  Value=zeros(3)
  Matrix Concatenate : Concatenate  Mode=Multidimensional array  ConcatenateDimension=2
  Matrix Concatenate1 : Concatenate  Mode=Multidimensional array  ConcatenateDimension=2
  Matrix Concatenate2 : Concatenate  Mode=Multidimensional array
  Matrix Multiply : Product  Multiplication=Matrix(*)
  Selector : Selector  NumberOfDimensions=2  InputPortWidth=3  IndexOptions=Index vector (dialog),Index vector (dialog)  Indices=1:3,1:3  OutputSizes=1,1
  Selector1 : Selector  NumberOfDimensions=2  InputPortWidth=3  IndexOptions=Index vector (dialog),Index vector (dialog)  Indices=1:3,4  OutputSizes=1,1
  vec2skew : Subsystem
  Ad : Outport
  wires:
  Selector1/1 -> vec2skew/1(x)
  Selector/1 -> Matrix Multiply/2, Matrix Concatenate1/2, Matrix Concatenate/1
  Constant/1 -> Matrix Concatenate/2
  vec2skew/1("[x]") -> Matrix Multiply/1
  Matrix Multiply/1 -> Matrix Concatenate1/1
  Matrix Concatenate1/1 -> Matrix Concatenate2/2
  Matrix Concatenate/1 -> Matrix Concatenate2/1
  Matrix Concatenate2/1 -> Ad/1
  T/1 -> Selector1/1, Selector/1

== system rr_arm_control/link_2/tform_inverse ==
  T : Inport
  Constant : Constant  Value=[0,0,0,1]
  Gain : Gain  Gain=-1
  Matrix Concatenate : Concatenate  Mode=Multidimensional array  ConcatenateDimension=2
  Matrix Concatenate1 : Concatenate  Mode=Multidimensional array
  Matrix Multiply : Product  Multiplication=Matrix(*)
  Reshape : Reshape  OutputDimensionality=Row vector (2-D)
  Selector : Selector  NumberOfDimensions=2  InputPortWidth=3  IndexOptions=Index vector (dialog),Index vector (dialog)  Indices=1:3,1:3  OutputSizes=1,1
  Selector1 : Selector  NumberOfDimensions=2  InputPortWidth=3  IndexOptions=Index vector (dialog),Index vector (dialog)  Indices=1:3,4  OutputSizes=1,1
  Transpose : Math  Operator=transpose
  Tinv : Outport
  wires:
  T/1 -> Selector1/1, Selector/1
  Selector/1 -> Transpose/1
  Transpose/1 -> Matrix Multiply/1, Matrix Concatenate/1
  Matrix Multiply/1 -> Gain/1
  Gain/1 -> Matrix Concatenate/2
  Matrix Concatenate/1 -> Matrix Concatenate1/1
  Constant/1 -> Reshape/1
  Matrix Concatenate1/1 -> Tinv/1
  Selector1/1 -> Matrix Multiply/2
  Reshape/1 -> Matrix Concatenate1/2

== system rr_arm_control/link_2/twist_adjoint ==
  V : Inport
  Constant : Constant  Value=zeros(3)
  Matrix Concatenate : Concatenate  Mode=Multidimensional array  ConcatenateDimension=2
  Matrix Concatenate1 : Concatenate  Mode=Multidimensional array  ConcatenateDimension=2
  Matrix Concatenate2 : Concatenate  Mode=Multidimensional array
  Selector : Selector  InputPortWidth=6  IndexOptions=Index vector (dialog)  Indices=1:3  OutputSizes=1
  Selector1 : Selector  InputPortWidth=6  IndexOptions=Index vector (dialog)  Indices=4:6  OutputSizes=1
  "[v]" : Subsystem
  "[w]" : Subsystem
  adV : Outport
  wires:
  Selector/1 -> "[w]"/1(x)
  Constant/1 -> Matrix Concatenate/2
  Matrix Concatenate1/1 -> Matrix Concatenate2/2
  Matrix Concatenate/1 -> Matrix Concatenate2/1
  Matrix Concatenate2/1 -> adV/1
  V/1 -> Selector1/1, Selector/1
  "[w]"/1("[x]") -> Matrix Concatenate1/2, Matrix Concatenate/1
  Selector1/1 -> "[v]"/1(x)
  "[v]"/1("[x]") -> Matrix Concatenate1/1

== system rr_arm_control/tform_adjoint/vec2skew ==
  x : Inport
  Constant : Constant  Value=0
  Demux : Demux  Outputs=3
  Gain : Gain  Gain=-1
  Gain1 : Gain  Gain=-1
  Gain2 : Gain  Gain=-1
  Matrix Concatenate : Concatenate  NumInputs=3  Mode=Multidimensional array  ConcatenateDimension=2
  Mux : Mux  Inputs=3
  Mux1 : Mux  Inputs=3
  Mux2 : Mux  Inputs=3
  "[x]" : Outport
  wires:
  Mux1/1 -> Matrix Concatenate/2
  Mux/1 -> Matrix Concatenate/1
  Mux2/1 -> Matrix Concatenate/3
  Matrix Concatenate/1 -> "[x]"/1
  Gain/1 -> Mux/3
  Gain1/1 -> Mux1/1
  Gain2/1 -> Mux2/2
  Constant/1 -> Mux/1, Mux1/2, Mux2/3
  x/1 -> Demux/1
  Demux/3 -> Gain1/1, Mux/2  "z"
  Demux/2 -> Mux2/1, Gain/1  "y"
  Demux/1 -> Gain2/1, Mux1/3  "x"

== system rr_arm_control/tform_adjoint1/vec2skew ==
  x : Inport
  Constant : Constant  Value=0
  Demux : Demux  Outputs=3
  Gain : Gain  Gain=-1
  Gain1 : Gain  Gain=-1
  Gain2 : Gain  Gain=-1
  Matrix Concatenate : Concatenate  NumInputs=3  Mode=Multidimensional array  ConcatenateDimension=2
  Mux : Mux  Inputs=3
  Mux1 : Mux  Inputs=3
  Mux2 : Mux  Inputs=3
  "[x]" : Outport
  wires:
  Mux1/1 -> Matrix Concatenate/2
  Mux/1 -> Matrix Concatenate/1
  Mux2/1 -> Matrix Concatenate/3
  Matrix Concatenate/1 -> "[x]"/1
  Gain/1 -> Mux/3
  Gain1/1 -> Mux1/1
  Gain2/1 -> Mux2/2
  Constant/1 -> Mux/1, Mux1/2, Mux2/3
  x/1 -> Demux/1
  Demux/3 -> Gain1/1, Mux/2  "z"
  Demux/2 -> Mux2/1, Gain/1  "y"
  Demux/1 -> Gain2/1, Mux1/3  "x"

== system rr_arm_control/damping_link_1/tform_adjoint/vec2skew ==
  x : Inport
  Constant : Constant  Value=0
  Demux : Demux  Outputs=3
  Gain : Gain  Gain=-1
  Gain1 : Gain  Gain=-1
  Gain2 : Gain  Gain=-1
  Matrix Concatenate : Concatenate  NumInputs=3  Mode=Multidimensional array  ConcatenateDimension=2
  Mux : Mux  Inputs=3
  Mux1 : Mux  Inputs=3
  Mux2 : Mux  Inputs=3
  "[x]" : Outport
  wires:
  Mux1/1 -> Matrix Concatenate/2
  Mux/1 -> Matrix Concatenate/1
  Mux2/1 -> Matrix Concatenate/3
  Matrix Concatenate/1 -> "[x]"/1
  Gain/1 -> Mux/3
  Gain1/1 -> Mux1/1
  Gain2/1 -> Mux2/2
  Constant/1 -> Mux/1, Mux1/2, Mux2/3
  x/1 -> Demux/1
  Demux/3 -> Gain1/1, Mux/2  "z"
  Demux/2 -> Mux2/1, Gain/1  "y"
  Demux/1 -> Gain2/1, Mux1/3  "x"

== system rr_arm_control/damping_link_2/tform_adjoint/vec2skew ==
  x : Inport
  Constant : Constant  Value=0
  Demux : Demux  Outputs=3
  Gain : Gain  Gain=-1
  Gain1 : Gain  Gain=-1
  Gain2 : Gain  Gain=-1
  Matrix Concatenate : Concatenate  NumInputs=3  Mode=Multidimensional array  ConcatenateDimension=2
  Mux : Mux  Inputs=3
  Mux1 : Mux  Inputs=3
  Mux2 : Mux  Inputs=3
  "[x]" : Outport
  wires:
  Mux1/1 -> Matrix Concatenate/2
  Mux/1 -> Matrix Concatenate/1
  Mux2/1 -> Matrix Concatenate/3
  Matrix Concatenate/1 -> "[x]"/1
  Gain/1 -> Mux/3
  Gain1/1 -> Mux1/1
  Gain2/1 -> Mux2/2
  Constant/1 -> Mux/1, Mux1/2, Mux2/3
  x/1 -> Demux/1
  Demux/3 -> Gain1/1, Mux/2  "z"
  Demux/2 -> Mux2/1, Gain/1  "y"
  Demux/1 -> Gain2/1, Mux1/3  "x"

== system rr_arm_control/gravity_link_1/tform_adjoint/vec2skew ==
  x : Inport
  Constant : Constant  Value=0
  Demux : Demux  Outputs=3
  Gain : Gain  Gain=-1
  Gain1 : Gain  Gain=-1
  Gain2 : Gain  Gain=-1
  Matrix Concatenate : Concatenate  NumInputs=3  Mode=Multidimensional array  ConcatenateDimension=2
  Mux : Mux  Inputs=3
  Mux1 : Mux  Inputs=3
  Mux2 : Mux  Inputs=3
  "[x]" : Outport
  wires:
  Mux1/1 -> Matrix Concatenate/2
  Mux/1 -> Matrix Concatenate/1
  Mux2/1 -> Matrix Concatenate/3
  Matrix Concatenate/1 -> "[x]"/1
  Gain/1 -> Mux/3
  Gain1/1 -> Mux1/1
  Gain2/1 -> Mux2/2
  Constant/1 -> Mux/1, Mux1/2, Mux2/3
  x/1 -> Demux/1
  Demux/3 -> Gain1/1, Mux/2  "z"
  Demux/2 -> Mux2/1, Gain/1  "y"
  Demux/1 -> Gain2/1, Mux1/3  "x"
